simulink model "W3prob3"  (R2020b)
settings: Solver=ode45  StartTime=0.0  StopTime=100  RelTol=1e-3
PreLoadFcn:
  | Vref=10;
  | V_lead_ini=20;
  | Pos_lead_ini=100;
  | Vset=30;
  | Tg=1.4;
  | V_follow_ini=30;
  | pos_follow_ini=0;
undefined symbols (not defined in the file or in its folder): sigbuilder_block
libraries: mpcadaslib x1
settings Model: Creator=deves  LastModifiedBy=deves

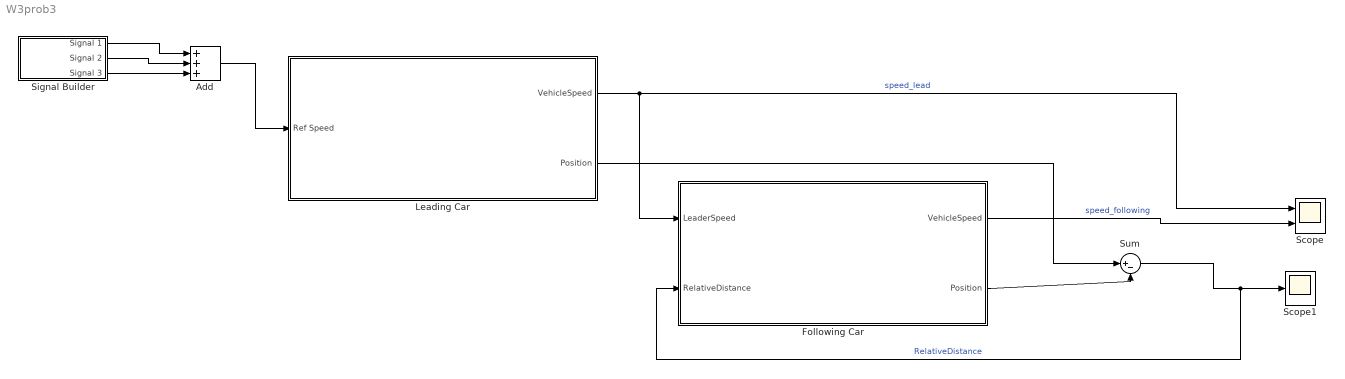
== system W3prob3 ==
  Add : Sum  Inputs=+++
  Following Car : Subsystem  mask{Pos=pos_follow_ini, Speed=V_follow_ini}
      mask prompts: Pos "InitialPosition"; Speed "InitialSpeed"
      mask TypeOptions Pos: InitialPosition/Value
      mask TypeOptions Speed: InitialSpeed/Value
  Leading Car : Subsystem  mask{Pos=Pos_lead_ini, Speed=V_lead_ini}
      mask prompts: Pos "InitialPosition"; Speed "InitialSpeed"
      mask TypeOptions Pos: InitialPosition/Value
      mask TypeOptions Speed: InitialSpeed/Value
  Scope : Scope  NumInputPorts=2
  Scope1 : Scope
  Signal Builder : Subsystem  Tag=STV Subsys  LoadFcn=sigbuilder_block('load');  StartFcn=sigbuilder_block('start');  StopFcn=sigbuilder_block('stop');  ClipboardFcn=sigbuilder_block('clipboard');  mask(Sigbuilder block){tuvar=[0:10]}
      mask help: Simulink:masks:SigbuilderBlock_MD
      mask init:
      | if ~strcmp(get_param(bdroot(gcbh),'SimulationStatus'),'stopped') tuvar = sigbuilder_block('maskInit'); end
      settings: CopyFcn=sigbuilder_block('copy');  DeleteFcn=sigbuilder_block('delete');  ModelCloseFcn=sigbuilder_block('modelClose');  PreSaveFcn=sigbuilder_block('preSave');  PauseFcn=sigbuilder_block('pause');  ContinueFcn=sigbuilder_block('continue');  NameChangeFcn=sigbuilder_block('namechange');  OpenFcn=sigbuilder_block('open',[5.4 30 1141.2 522.6 ]);  CloseFcn=sigbuilder_block('close');
      mask Display: plot(0, 0, 100, 100,[2, 2, 32, 32, 2], [68, 8, 8, 68, 68],[32, 2], [38, 38], [32, 19, 2],[53, 60, 44], [32, 17, 17, 2],[16, 16, 31, 31]);txt = getActiveGroup(gcbh);text(2, 100, txt,'verticalAlignment', 'top');
  Sum : Sum  Inputs=|+-
  wires:
  Add/1 -> Leading Car/1(Ref Speed)
  Leading Car/1(VehicleSpeed) -> Scope/1, Following Car/1(LeaderSpeed)  "speed_lead"
  Leading Car/2(Position) -> Sum/1
  Following Car/2(Position) -> Sum/2
  Sum/1 -> Following Car/2(RelativeDistance), Scope1/1  "RelativeDistance"
  Following Car/1(VehicleSpeed) -> Scope/2  "speed_following"
  Signal Builder/1(Signal 1) -> Add/1
  Signal Builder/2(Signal 2) -> Add/2
  Signal Builder/3(Signal 3) -> Add/3

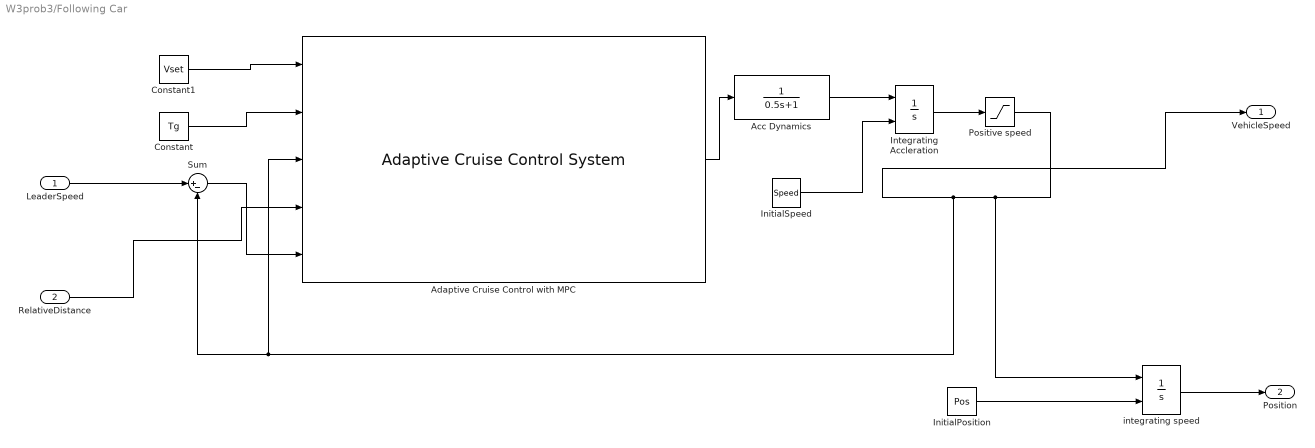
== system W3prob3/Following Car ==
  LeaderSpeed : Inport
  RelativeDistance : Inport  Port=2
  Acc Dynamics : TransferFcn  Denominator=[0.5 1 ]
  "Adaptive Cruise Control with MPC " : mpcadaslib/Adaptive Cruise Control System  EgoModel=tf(1,[0.5,1,0])  InitialEgoVelocity=30  DefaultSpacing=10  MaxVelocity=50  MinAcceleration=-3  amin_ext=off  MaxAcceleration=2  amax_ext=off  Ts=0.5  PredictionHorizon=300  ControllerBehavior=0.45  suboptimal=off  maxiter=10  datatypeopt=double  optmode=off  trackmode=off  mask(Adaptive cruise control (ACC) system){}
      mask Display: image('C:\Users\deves\OneDrive\Pictures\adaptive_detail01.jpg'); % Use "Edit Image" on toolstrip to change.
  Constant : Constant  Value=Tg
  Constant1 : Constant  Value=Vset
  InitialPosition : Constant  Value=Pos
  InitialSpeed : Constant  Value=Speed
  Integrating Accleration : Integrator  InitialConditionSource=external
  Positive speed : Saturate  UpperLimit=inf  LowerLimit=0
  Sum : Sum  Inputs=|+-
  integrating speed : Integrator  InitialConditionSource=external
  VehicleSpeed : Outport
  Position : Outport  Port=2
  wires:
  InitialPosition/1 -> integrating speed/2
  LeaderSpeed/1 -> Sum/1
  Integrating Accleration/1 -> Positive speed/1
  Acc Dynamics/1 -> Integrating Accleration/1
  Positive speed/1 -> VehicleSpeed/1, "Adaptive Cruise Control with MPC "/3, Sum/2, integrating speed/1
  "Adaptive Cruise Control with MPC "/1 -> Acc Dynamics/1
  InitialSpeed/1 -> Integrating Accleration/2
  integrating speed/1 -> Position/1
  Sum/1 -> "Adaptive Cruise Control with MPC "/5
  RelativeDistance/1 -> "Adaptive Cruise Control with MPC "/4
  Constant/1 -> "Adaptive Cruise Control with MPC "/2
  Constant1/1 -> "Adaptive Cruise Control with MPC "/1

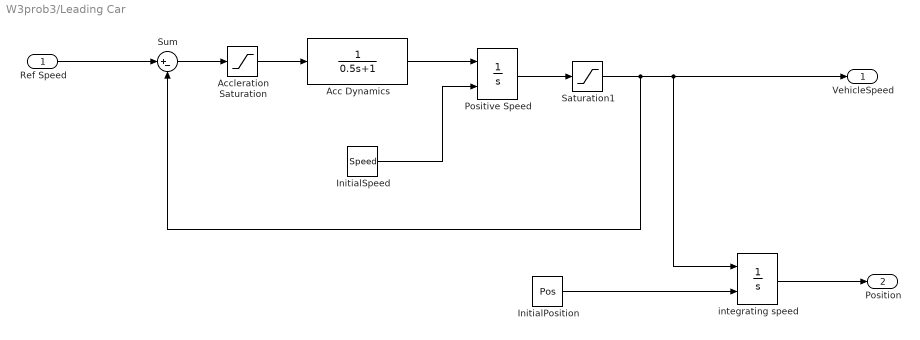
== system W3prob3/Leading Car ==
  Ref Speed : Inport
  Acc Dynamics : TransferFcn  Denominator=[0.5 1 ]
  Accleration Saturation : Saturate  UpperLimit=2  LowerLimit=-3
  InitialPosition : Constant  Value=Pos
  InitialSpeed : Constant  Value=Speed
  Positive Speed : Integrator  InitialConditionSource=external
  Saturation1 : Saturate  UpperLimit=inf  LowerLimit=0
  Sum : Sum  Inputs=|+-
  integrating speed : Integrator  InitialConditionSource=external
  VehicleSpeed : Outport
  Position : Outport  Port=2
  wires:
  integrating speed/1 -> Position/1
  InitialSpeed/1 -> Positive Speed/2
  Accleration Saturation/1 -> Acc Dynamics/1
  Saturation1/1 -> Sum/2, VehicleSpeed/1, integrating speed/1
  Acc Dynamics/1 -> Positive Speed/1
  Sum/1 -> Accleration Saturation/1
  Positive Speed/1 -> Saturation1/1
  Ref Speed/1 -> Sum/1
  InitialPosition/1 -> integrating speed/2

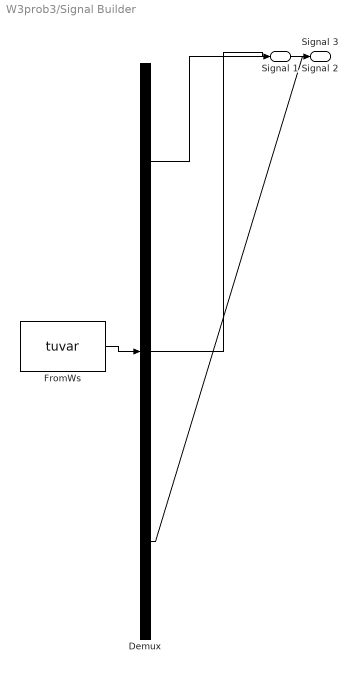
== system W3prob3/Signal Builder ==
  Demux : Demux  Tag=STV Demux  Outputs=3
      settings: DisplayOption=none
  FromWs : FromWorkspace  Tag=STV FromWs  VariableName=tuvar
      SigBuilderData=|
      | common.afterFinalStr = 'Extrapolate'
      | common.sampleTime = 0
      | dataSet.timeRange = [0 100]
      | dataSet.name = 'Group 1'
      | sbobj.Groups.Name = 'Group 1'
      | sbobj.Groups.Signals(1).Name = 'Signal 1'
      | sbobj.Groups.Signals(1).XData = [0 100]
      | sbobj.Groups.Signals(1).YData = [10 10]
      | sbobj.Groups.Signals(2).Name = 'Signal 2'
      | sbobj.Groups.Signals(2).XData = [0 30 30 100]
      | sbobj.Groups.Signals(2).YData = [0 0 10 10]
      | sbobj.Groups.Signals(3).Name = 'Signal 3'
      | sbobj.Groups.Signals(3).XData = [0 60 60 100]
      | sbobj.Groups.Signals(3).YData = [0 0 10 10]
      | sbobj.Groups.TimeRange = [0 100]
  Signal 1 : Outport  Tag=STV Outport
  Signal 2 : Outport  Tag=STV Outport  Port=2
  Signal 3 : Outport  Tag=STV Outport  Port=3
  wires:
  FromWs/1 -> Demux/1
  Demux/1 -> Signal 1/1
  Demux/2 -> Signal 2/1
  Demux/3 -> Signal 3/1
